simulink model "hw4_1b_ii_model_force_tracking"  (R2022b)
settings: Solver=VariableStepAuto  StartTime=0.0  StopTime=10.0  RelTol=1e-3
undefined symbols (not defined in the file): b
settings Model: Creator=gaura  LastModifiedBy=gaura

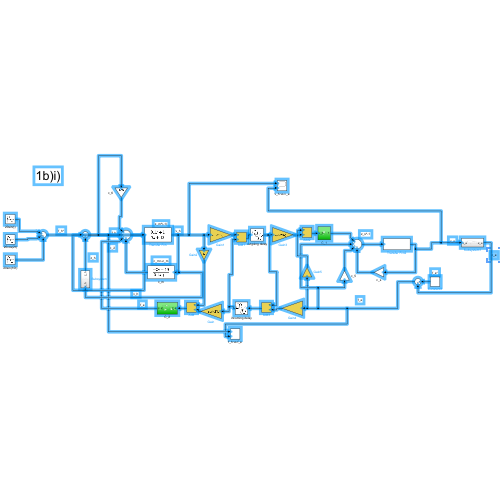
[thumbnail: Simulink's stored preview of the top-level diagram]
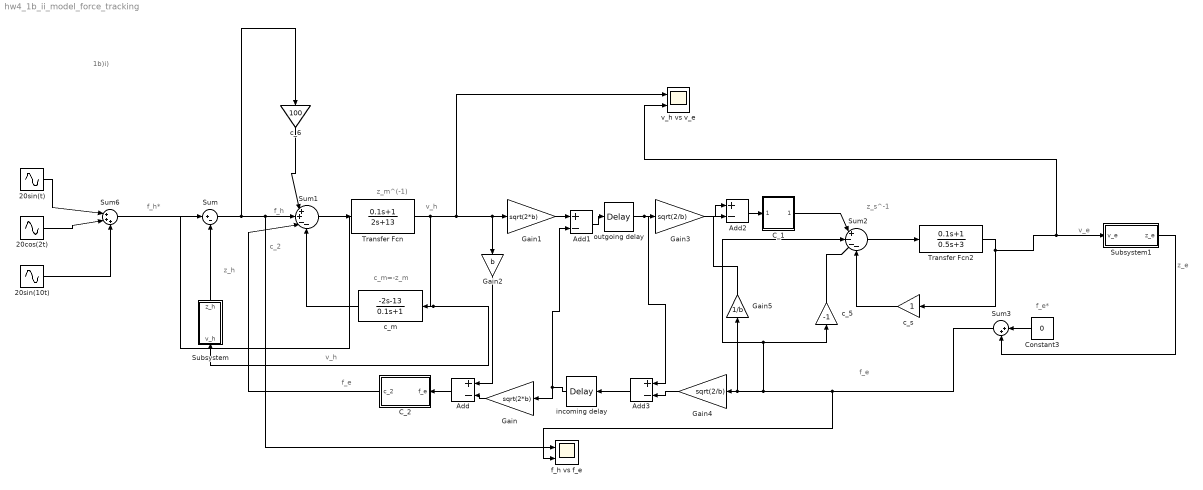
== system hw4_1b_ii_model_force_tracking ==
  note: v_e
  note: f_e*
  note: v_h
  note: z_s^-1
  note: c_2
  note: f_h*
  note: c_m=-z_m
  note: v_h
  note: f_h
  note: z_m^(-1)
  note: 1b)i)
  note: f_e
  note: f_e
  note: z_h
  note: z_e
  20cos(2t) : Sin  Amplitude=20  Frequency=2  Phase=pi/2  SampleTime=0
  20sin(10t) : Sin  Amplitude=20  Frequency=10  SampleTime=0
  20sin(t) : Sin  Amplitude=20  SampleTime=0
  Add{,1..3} (4 alike) : Sum  Inputs=+-
  C_1 : Subsystem
  C_2 : Subsystem
  Constant3 : Constant  Value=0
  Gain : Gain  Gain=sqrt(2*b)
  Gain1 : Gain  Gain=sqrt(2*b)
  Gain2 : Gain  Gain=b
  Gain3 : Gain  Gain=sqrt(2/b)
  Gain4 : Gain  Gain=sqrt(2/b)
  Gain5 : Gain  Gain=1/b
  Subsystem : Subsystem
  Subsystem1 : Subsystem
  Sum : Sum  Inputs=|+-
  Sum1 : Sum  Inputs=|++--
  Sum2 : Sum  Inputs=|+---
  Sum3 : Sum  Inputs=|++
  Sum6 : Sum  Inputs=|+++
  Transfer Fcn : TransferFcn  Numerator=[0.1 1]  Denominator=[2 13]
  Transfer Fcn2 : TransferFcn  Numerator=[0.1 1]  Denominator=[0.5 3]
  c_5 : Gain  Gain=-1
  c_6 : Gain  Gain=100
  c_m : TransferFcn  Numerator=[-2 -13]  Denominator=[0.1 1]
  c_s : Gain
  f_h vs f_e : Scope  NumInputPorts=2
  incoming delay : TransportDelay  DelayTime=0.1
  outgoing delay : TransportDelay  DelayTime=0.1
  v_h vs v_e : Scope  NumInputPorts=2
  wires:
  C_1/1(Output) -> Sum2/1
  Transfer Fcn/1 -> v_h vs v_e/1, Gain2/1, Gain1/1, Subsystem/1(v_h), c_m/1
  Gain2/1 -> Add/1
  C_2/1(c_2) -> Sum1/3
  outgoing delay/1 -> Add3/1, Gain3/1
  Gain3/1 -> Add2/1
  Gain4/1 -> Add3/2
  Sum/1 -> f_h vs f_e/1, Sum1/2, c_6/1
  Gain5/1 -> Add2/2
  Sum1/1 -> Transfer Fcn/1
  Gain/1 -> Add/2
  20cos(2t)/1 -> Sum6/2
  Constant3/1 -> Sum3/1
  Subsystem/1(z_h) -> Sum/2
  Add3/1 -> incoming delay/1
  Add1/1 -> outgoing delay/1
  incoming delay/1 -> Add1/2, Gain/1
  Gain1/1 -> Add1/1
  Transfer Fcn2/1 -> v_h vs v_e/2, Subsystem1/1(v_e), c_s/1
  Add2/1 -> C_1/1(v_h)
  Sum3/1 -> f_h vs f_e/2, Gain4/1, Gain5/1, c_5/1, Sum2/2
  c_s/1 -> Sum2/4
  20sin(t)/1 -> Sum6/1
  c_5/1 -> Sum2/3
  c_6/1 -> Sum1/1
  Sum2/1 -> Transfer Fcn2/1
  20sin(10t)/1 -> Sum6/3
  Sum6/1 -> Sum/1
  c_m/1 -> Sum1/4
  Subsystem1/1(z_e) -> Sum3/2
  Add/1 -> C_2/1(f_e)

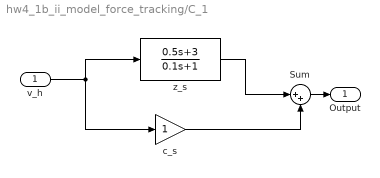
== system hw4_1b_ii_model_force_tracking/C_1 ==
  v_h : Inport
  Sum : Sum  Inputs=|++
  c_s : Gain
  z_s : TransferFcn  Numerator=[0.5 3]  Denominator=[0.1 1]
  Output : Outport
  wires:
  z_s/1 -> Sum/1
  v_h/1 -> c_s/1, z_s/1
  Sum/1 -> Output/1
  c_s/1 -> Sum/2

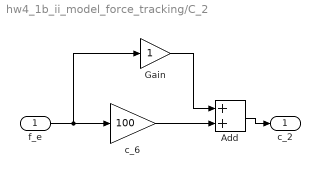
== system hw4_1b_ii_model_force_tracking/C_2 ==
  f_e : Inport
  Add : Sum
  Gain : Gain
  c_6 : Gain  Gain=100
  c_2 : Outport
  wires:
  f_e/1 -> Gain/1, c_6/1
  Gain/1 -> Add/1
  c_6/1 -> Add/2
  Add/1 -> c_2/1

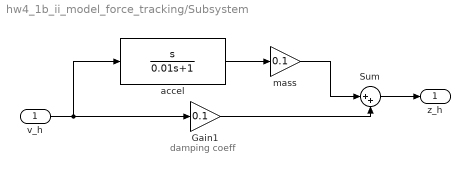
== system hw4_1b_ii_model_force_tracking/Subsystem ==
  note: damping coeff
  v_h : Inport
  Gain1 : Gain  Gain=0.1
  Sum : Sum  Inputs=|++
  accel : TransferFcn  Numerator=[1 0]  Denominator=[0.01 1]
  mass : Gain  Gain=0.1
  z_h : Outport
  wires:
  v_h/1 -> Gain1/1, accel/1
  accel/1 -> mass/1
  mass/1 -> Sum/1
  Sum/1 -> z_h/1
  Gain1/1 -> Sum/2

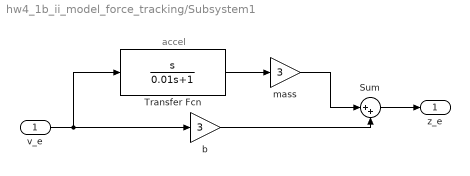
== system hw4_1b_ii_model_force_tracking/Subsystem1 ==
  note: accel
  v_e : Inport
  Sum : Sum  Inputs=|++
  Transfer Fcn : TransferFcn  Numerator=[1 0]  Denominator=[0.01 1]
  b : Gain  Gain=3
  mass : Gain  Gain=3
  z_e : Outport
  wires:
  mass/1 -> Sum/1
  Sum/1 -> z_e/1
  Transfer Fcn/1 -> mass/1
  b/1 -> Sum/2
  v_e/1 -> b/1, Transfer Fcn/1
